simulink model "Exercise3_simulink"  (R2023b)
settings: Solver=VariableStepAuto  StartTime=0.0  StopTime=t_final  RelTol=1e-3
values from neighbouring files (symbols this model uses):
  F = Opt_flow    [call_RTO.m]    (also in minCostFunction.m = x(1); nonlinearcon.m = x(1); s_func3.m = u(1))
  kla = Opt_kla    [call_RTO.m]    (also in minCostFunction.m = x(3); nonlinearcon.m = x(3); s_func3.m = u(4))
  par = [Y_xs,micro_max,K_s,K_o,O_sat]    [call_RTO.m]
  S_f = 10    [call_RTO.m]    (also in nonlinearcon.m; s_func3.m = u(2))
  temp = Opt_temp    [call_RTO.m]    (also in s_func3.m = u(3))
  xinit = [x_init s_init o_init]    [call_RTO.m]
settings Model: Creator=s223593  LastModifiedBy=s223593

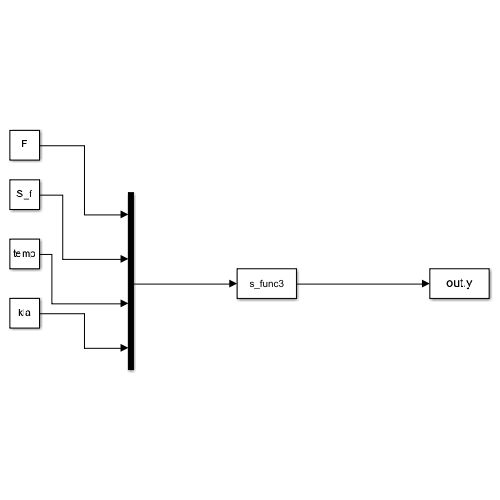
[thumbnail: Simulink's stored preview of the top-level diagram]
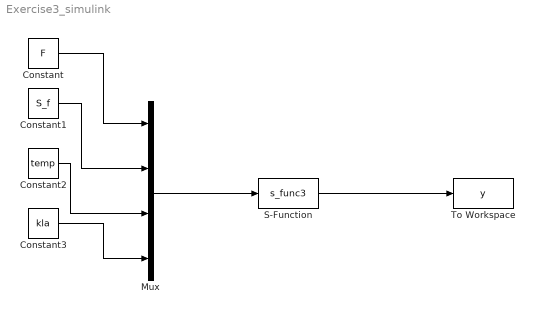
== system Exercise3_simulink ==
  Constant : Constant  Value=F
  Constant1 : Constant  Value=S_f
  Constant2 : Constant  Value=temp
  Constant3 : Constant  Value=kla
  Mux : Mux
  S-Function : S-Function  FunctionName=s_func3  Parameters=xinit,par  SFunctionDeploymentMode=off  EnableBusSupport=off
  To Workspace : ToWorkspace  VariableName=y  SampleTime=-1
  wires:
  Constant/1 -> Mux/1
  Constant1/1 -> Mux/2
  Constant2/1 -> Mux/3
  Constant3/1 -> Mux/4
  Mux/1 -> S-Function/1
  S-Function/1 -> To Workspace/1
